simulink model "PID_1"  (R2019a)
settings: Solver=VariableStepAuto  StartTime=0.0  StopTime=50  RelTol=1e-3
undefined symbols (not defined in the file): J, Ke_Phi, Km_Phi, La, Ra
libraries: simulink x1
settings Model: Creator=Chi Tuyen  LastModifiedBy=Chi Tuyen
settings DebuggingCC: ArithmeticOperatorsInVariantConditions=warning

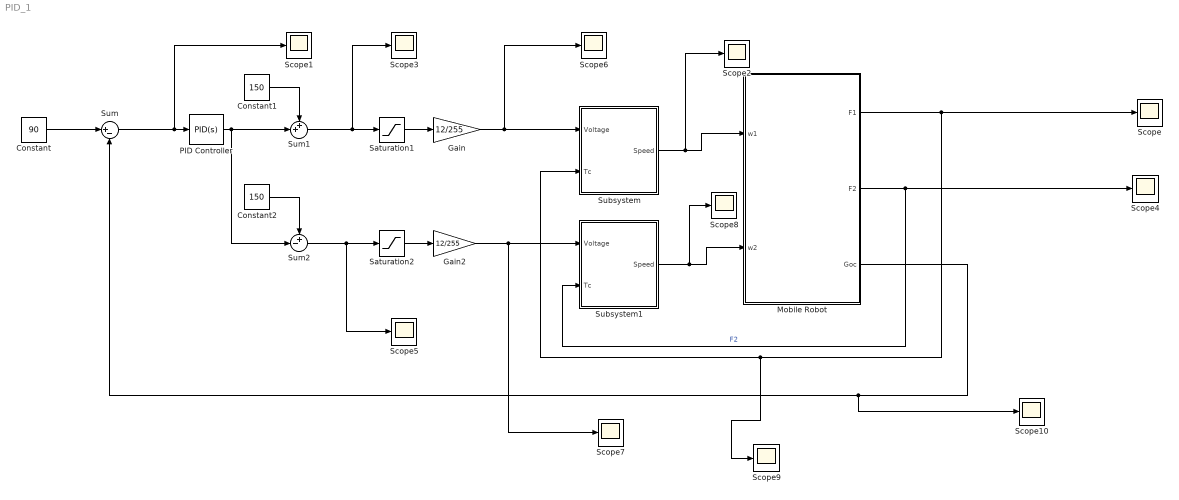
== system PID_1 ==
  Constant : Constant  Value=90
  Constant1 : Constant  Value=150
  Constant2 : Constant  Value=150
  Gain : Gain  Gain=12/255
  Gain2 : Gain  Gain=12/255
  Mobile Robot : Subsystem
  PID Controller : simulink/Continuous/PID Controller  Controller=PID  Form=Parallel  TimeDomain=Continuous-time  SampleTime=-1  IntegratorMethod=Forward Euler  FilterMethod=Forward Euler  ControllerParametersSource=internal  P=1.5  I=5  D=10  UseFilter=on  N=1  TunerSelectOption=Transfer Function Based (PID Tuner App)  InitialConditionSource=internal  InitialConditionForIntegrator=0  InitialConditionForFilter=0  DifferentiatorICPrevScaledInput=0  ExternalReset=none  TrackingMode=off  Kt=1  LimitOutput=off  UpperSaturationLimit=inf  LowerSaturationLimit=-inf  LinearizeAsGain=on  AntiWindupMode=none  Kb=1  POutMin=[]  POutMax=[]  IOutMin=[]  IOutMax=[]  DOutMin=[]  DOutMax=[]  NOutMin=[]  NOutMax=[]  SumOutMin=[]  SumOutMax=[]  SaturationOutMin=[]  SaturationOutMax=[]  PParamMin=[]  PParamMax=[]  IParamMin=[]  IParamMax=[]  DParamMin=[]  DParamMax=[]  NParamMin=[]  NParamMax=[]  KbParamMin=[]  KbParamMax=[]  KtParamMin=[]  KtParamMax=[]  KbOutMin=[]  KbOutMax=[]  KtOutMin=[]  KtOutMax=[]  IntegratorOutMin=[]  IntegratorOutMax=[]  FilterOutMin=[]  FilterOutMax=[]  SumI1OutMin=[]  SumI1OutMax=[]  SumI2OutMin=[]  SumI2OutMax=[]  SumI3OutMin=[]  SumI3OutMax=[]  SumI4OutMin=[]  SumI4OutMax=[]  SumDOutMin=[]  SumDOutMax=[]  DifferentiatorOutMin=[]  DifferentiatorOutMax=[]  FilterDiffOutCoefMin=[]  FilterDiffOutCoefMax=[]  ReciprocalOutMin=[]  ReciprocalOutMax=[]  SumDenOutMin=[]  SumDenOutMax=[]  SumNumOutMin=[]  SumNumOutMax=[]  DivideOutMin=[]  DivideOutMax=[]  IntegratorContinuousStateAttributes=''  IntegratorStateMustResolveToSignalObject=off  IntegratorRTWStateStorageClass=Auto  FilterContinuousStateAttributes=''  FilterStateMustResolveToSignalObject=off  FilterRTWStateStorageClass=Auto  ParallelPVariant=InternalParameters  IdealPVariant=Disabled  IVariant=InternalParameters  DVariant=InternalParameters  IntegratorVariant=Continuous  SatVariant=Disabled  AWVariant=Passthrough  PCopyVariant=Disabled  TRVariant=Disabled  FdbkBlocksVariant=Forward  IdealPFdbkVariant=Disabled  SatFdbkVariant=Disabled  DerivativeFilterVariant=ContFilter  NVariant=InternalParameters  NCopyVariant=Disabled  FilterICVariant=InternalICsFilter  IntegratorICVariant=InternalICs  ExternalResetVariant=Disabled  TRSumVariant=Passthrough  SumFdbkVariant=Disabled  SumVariant=Sum_PID
  Saturation1 : Saturate  UpperLimit=230  LowerLimit=0
  Saturation2 : Saturate  UpperLimit=230  LowerLimit=0
  Scope{,1..10} (11 alike) : Scope
  Subsystem : Subsystem
  Subsystem1 : Subsystem
  Sum : Sum  Inputs=|+-
  Sum1 : Sum  Inputs=++|
  Sum2 : Sum  Inputs=+-|
  wires:
  Constant/1 -> Sum/1
  Sum/1 -> PID Controller/1, Scope1/1
  Mobile Robot/1(F1) -> Scope9/1, Subsystem/2("Tc "), Scope/1
  Subsystem1/1("Speed ") -> Scope8/1, Mobile Robot/2(w2)
  Mobile Robot/2(F2) -> Subsystem1/2("Tc "), Scope4/1  "F2"
  Subsystem/1("Speed ") -> Scope2/1, Mobile Robot/1(w1)
  Saturation1/1 -> Gain/1
  Gain/1 -> Scope6/1, Subsystem/1("Voltage ")
  Saturation2/1 -> Gain2/1
  Gain2/1 -> Scope7/1, Subsystem1/1("Voltage ")
  Sum1/1 -> Scope3/1, Saturation1/1
  Constant1/1 -> Sum1/1
  PID Controller/1 -> Sum2/2, Sum1/2
  Sum2/1 -> Scope5/1, Saturation2/1
  Constant2/1 -> Sum2/1
  Mobile Robot/3("Goc ") -> Scope10/1, Sum/2

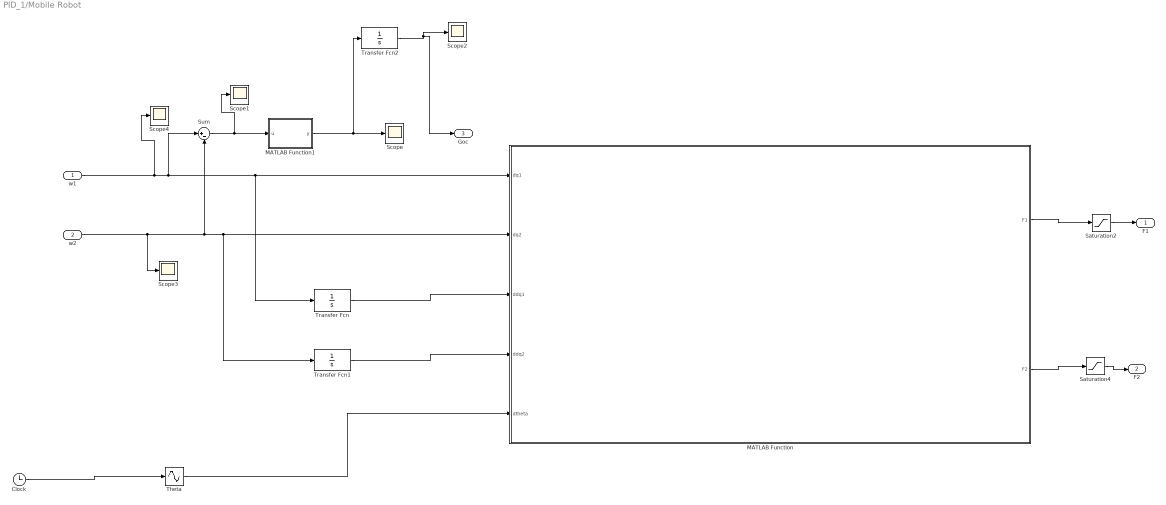
== system PID_1/Mobile Robot ==
  w1 : Inport
  w2 : Inport  Port=2
  Clock : Clock
      settings: Decimation=5
  MATLAB Function : MATLAB Function  TreatAsAtomicUnit=on
  MATLAB Function1 : MATLAB Function  TreatAsAtomicUnit=on
  Saturation2 : Saturate
  Saturation4 : Saturate
  Scope{,1..4} (5 alike) : Scope
  Sum : Sum  Inputs=|+-
  Theta : Sin  TimeSource=Use external signal  Frequency=60  Phase=30  SampleTime=0
  Transfer Fcn : TransferFcn  Denominator=[1 0]
  Transfer Fcn1 : TransferFcn  Denominator=[1 0]
  Transfer Fcn2 : TransferFcn  Denominator=[1 0]
  F1 : Outport
  F2 : Outport  Port=2
  "Goc " : Outport  Port=3
  wires:
  Clock/1 -> Theta/1
  Theta/1 -> MATLAB Function/5(dtheta)
  Saturation2/1 -> F1/1
  MATLAB Function/1(F1) -> Saturation2/1
  MATLAB Function/2(F2) -> Saturation4/1
  Saturation4/1 -> F2/1
  Sum/1 -> MATLAB Function1/1(u), Scope1/1
  Transfer Fcn/1 -> MATLAB Function/3(ddq1)
  Transfer Fcn1/1 -> MATLAB Function/4(ddq2)
  MATLAB Function1/1(y) -> Transfer Fcn2/1, Scope/1
  Transfer Fcn2/1 -> "Goc "/1, Scope2/1
  w1/1 -> Scope4/1, Transfer Fcn/1, MATLAB Function/1(dq1), Sum/1
  w2/1 -> Scope3/1, Sum/2, Transfer Fcn1/1, MATLAB Function/2(dq2)

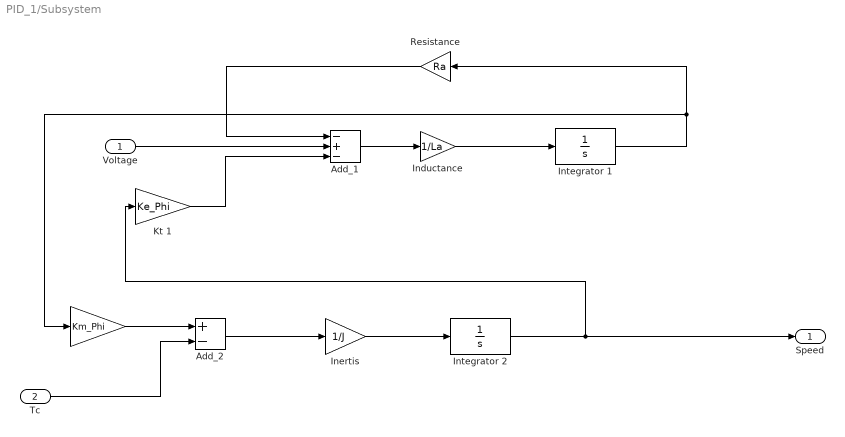
== system PID_1/Subsystem ==
  "Voltage " : Inport
  "Tc " : Inport  Port=2
  " " : Gain  Gain=Km_Phi
  "Add_1 " : Sum  Inputs=-+-
  "Add_2 " : Sum  Inputs=+-
  "Inductance " : Gain  Gain=1/La
  "Inertis " : Gain  Gain=1/J
  "Integrator 1 " : TransferFcn  Denominator=[1 0]
  "Integrator 2 " : TransferFcn  Denominator=[1 0]
  Kt 1 : Gain  Gain=Ke_Phi
  Resistance : Gain  Gain=Ra
  "Speed " : Outport
  wires:
  "Inductance "/1 -> "Integrator 1 "/1
  "Integrator 1 "/1 -> Resistance/1, " "/1
  "Inertis "/1 -> "Integrator 2 "/1
  "Integrator 2 "/1 -> "Speed "/1, Kt 1/1
  " "/1 -> "Add_2 "/1
  "Add_2 "/1 -> "Inertis "/1
  "Add_1 "/1 -> "Inductance "/1
  "Voltage "/1 -> "Add_1 "/2
  Resistance/1 -> "Add_1 "/1
  Kt 1/1 -> "Add_1 "/3
  "Tc "/1 -> "Add_2 "/2

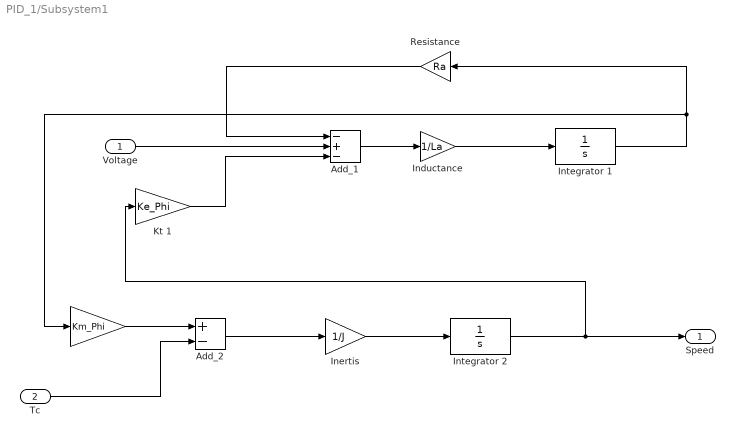
== system PID_1/Subsystem1 ==
  "Voltage " : Inport
  "Tc " : Inport  Port=2
  " " : Gain  Gain=Km_Phi
  "Add_1 " : Sum  Inputs=-+-
  "Add_2 " : Sum  Inputs=+-
  "Inductance " : Gain  Gain=1/La
  "Inertis " : Gain  Gain=1/J
  "Integrator 1 " : TransferFcn  Denominator=[1 0]
  "Integrator 2 " : TransferFcn  Denominator=[1 0]
  Kt 1 : Gain  Gain=Ke_Phi
  Resistance : Gain  Gain=Ra
  "Speed " : Outport
  wires:
  "Tc "/1 -> "Add_2 "/2
  Kt 1/1 -> "Add_1 "/3
  Resistance/1 -> "Add_1 "/1
  "Voltage "/1 -> "Add_1 "/2
  "Add_1 "/1 -> "Inductance "/1
  "Add_2 "/1 -> "Inertis "/1
  " "/1 -> "Add_2 "/1
  "Integrator 2 "/1 -> Kt 1/1, "Speed "/1
  "Inertis "/1 -> "Integrator 2 "/1
  "Integrator 1 "/1 -> " "/1, Resistance/1
  "Inductance "/1 -> "Integrator 1 "/1

== matlab function PID_1/Mobile Robot/MATLAB Function1 ==
  data: u input; y output
function y = fcn(u)
a=u*0.066;
b=2*0.12;
y = a/b;

== matlab function PID_1/Mobile Robot/MATLAB Function ==
  data: dq1 input; dq2 input; ddq1 input; ddq2 input; dtheta input; F1 output; F2 output
function [F1,F2]= fcn(dq1,dq2,ddq1,ddq2,dtheta)
IW=0.00009;
R=0.001;
mc=1;
mw=0.9;
L=12;
d=5;
Ic=2;
Im=0.001;

dq=[dq1;dq2];
ddq=[ddq1;ddq2];
m=mc+2*mw;
I=Ic+mc*d^2+2*mw*L^2+2*Im;

M=[IW+(R^2)*(m*L^2+I)/(4*L),(R^2)*(m*L^2-I)/(4*L);
    (R^2)*(m*L^2-I)/(4*L) ,IW+(R^2)*(m*L^2+I)/(4*L)];
    
V=[0, (R^2)*(mc*dtheta)/(2*L);
  -(R^2)*(mc*dtheta)/(2*L),0];

F=M*ddq+V*dq;
F1=F(1,1);
F2=F(2,1);
